simulink model "mlf_shiftreg"  (R2015b)
settings: Solver=FixedStepDiscrete  SolverMode=SingleTasking  StartTime=0.0  StopTime=10  RelTol=1e-3
libraries: simulink x1
settings Model: DataTypeOverride=Off  Creator=amatsumo  LastModifiedBy=amatsumo
settings DataIOCC: SaveFormat=Array  SignalLoggingSaveFormat=ModelDataLogs  SaveOutput=off  SignalLogging=off  SaveTime=off
settings OptimizationCC: BlockReduction=off  ConditionallyExecuteInputs=off  DefaultParameterBehavior=Inlined  ExpressionDepthLimit=2147483647
settings DebuggingCC: AlgebraicLoopMsg=error  UnderspecifiedInitializationDetection=Classic  MergeDetectMultiDrivingBlocksExec=none  SolverPrmCheckMsg=warning  SingleTaskRateTransMsg=error  FcnCallInpInsideContextMsg=UseLocalSettings  StateNameClashWarn=warning
settings HardwareCC: ProdBitPerPointer=32  ProdLargestAtomicFloat=None  ProdIntDivRoundTo=Undefined  ProdEndianess=Unspecified  ProdWordSize=32  ProdHWDeviceType=ASIC/FPGA->ASIC/FPGA  ProdEqTarget=off
settings GRTTargetCC: GeneratePreprocessorConditionals=Disable all  CombineOutputUpdateFcns=off  GRTInterface=on
settings ConfigComp: CovModelRefEnable=Off  CovSFcnEnable=off

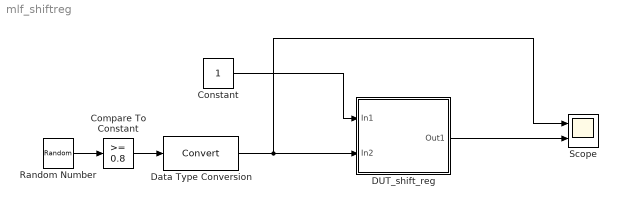
== system mlf_shiftreg ==
  Compare To Constant : simulink/Logic and Bit Operations/Compare To Constant  relop=>=  const=0.8  OutDataTypeStr=uint8
  Constant : Constant  OutDataTypeStr=boolean  SampleTime=-1
  DUT_shift_reg : Subsystem
  Data Type Conversion : DataTypeConversion
  Random Number : RandomNumber  SampleTime=0.1
  Scope : Scope  NumInputPorts=2
  wires:
  Random Number/1 -> Compare To Constant/1
  Constant/1 -> DUT_shift_reg/1(In1)
  DUT_shift_reg/1(Out1) -> Scope/2
  Data Type Conversion/1 -> Scope/1, DUT_shift_reg/2(In2)
  Compare To Constant/1 -> Data Type Conversion/1

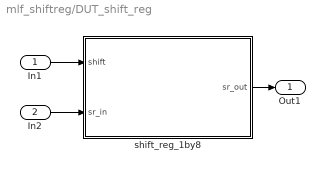
== system mlf_shiftreg/DUT_shift_reg ==
  In1 : Inport
  In2 : Inport  Port=2
  shift_reg_1by8 : MATLAB Function  TreatAsAtomicUnit=on
  Out1 : Outport
  wires:
  In2/1 -> shift_reg_1by8/2(sr_in)
  In1/1 -> shift_reg_1by8/1(shift)
  shift_reg_1by8/1(sr_out) -> Out1/1

== matlab function mlf_shiftreg/DUT_shift_reg/shift_reg_1by8 ==
  settings: fimath=hdlfimath;
  data: shift input boolean; sr_out output fixdt(0,1,0); sr_in input fixdt(0,1,0)
function sr_out = fcn(shift, sr_in)
%shift register

% 状態量の定義
persistent sr;
if isempty(sr)
    sr = fi(0, 0, 8, 0);
end

% MSBを出力
sr_out = getmsb(sr);

% Dataを遅延
if (shift)
    sr = bitconcat(bitsliceget(sr, 7, 1), sr_in);
end
